simulink model "Adder_1"  (R2018a)
settings: Solver=VariableStepAuto  StartTime=0.0  StopTime=10.0  RelTol=1e-3
settings Model: Creator=midog  LastModifiedBy=midog

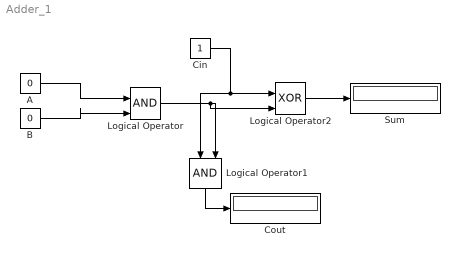
== system Adder_1 ==
  A : Constant  Value=0
  B : Constant  Value=0
  Cin : Constant
  Cout : Display
  Logical Operator : Logic  IconShape=distinctive  AllPortsSameDT=off  OutDataTypeStr=boolean
  Logical Operator1 : Logic  IconShape=distinctive  AllPortsSameDT=off  OutDataTypeStr=boolean
  Logical Operator2 : Logic  Operator=XOR  IconShape=distinctive  AllPortsSameDT=off  OutDataTypeStr=boolean
  Sum : Display
  wires:
  A/1 -> Logical Operator/1
  B/1 -> Logical Operator/2
  Logical Operator/1 -> Logical Operator2/2, Logical Operator1/2
  Cin/1 -> Logical Operator1/1, Logical Operator2/1
  Logical Operator2/1 -> Sum/1
  Logical Operator1/1 -> Cout/1
